simulink model "TorqueVect_HIL_CAN"  (R2022a)
settings: Solver=VariableStepAuto  StartTime=0.0  StopTime=300  RelTol=1e-3
PreLoadFcn:
  | run('Parameters\FSE_Parameters.m')
values from neighbouring files (symbols this model uses):
  Kd = 0;')    [open_carmaker_gui.m]
  Ki = 0    [open_carmaker_gui.m]
undefined symbols (not defined in the file or in its folder): BRegenEnabledButton, canChannel, CyalphaLookUp, efficiency, Fz_curve, Fz_scaling_long, gearR, izz, jw, kd, ki, Kp, kp, l_f, l_r, lambda, m, Mz_max, N, N_lat, N_long, P_max, pid_kd_lat, pid_kd_long, pid_ki_lat, pid_ki_long, pid_kp_lat, pid_kp_long, R_max, rw, steerR, T_i_max, TC_Decr_Gas, TC_Derivative, TC_Incr_Gas, TC_On, TC_Relay_Off, TC_Relay_On, tireCornerStiffness, Ts, TV_On, TV_Override, velocity_lookup, velocity_lookup_lat, y_ref, yrr_scaling
libraries: simulink x218, slpidlib x135, CarMaker4SL x73, TractionControlLibrary x13, canmsglib x11, canlib x10, TorqueVectoringLibrary x6, simulink_extras x4, PedalConversionLibrary x3, PowerControlLibrary x1
(part 17 of 26)

== system TorqueVect_HIL_CAN/CarMaker/IPG Vehicle/PowerTrain/PTControl Example/PTControl_ALL_CTRL_VC_REGEN/Subsystem/TC/TractionControlRL ==
  rSlipTarget : Inport
  rSlipMeasured : Inport  Port=2
  BEnableTC : Inport  Port=3
  P_TC : Inport  Port=4
  D_TC : Inport  Port=5
  I_TC : Inport  Port=6
  FF_TC : Inport  Port=7
  MMotorMax : Inport  Port=8
  MMotorRequest : Inport  Port=9
  If : If  NumInputs=2  IfExpression=u1 <= 0  ElseIfExpressions=u2 > u1
  If Action Subsystem : Subsystem  TreatAsAtomicUnit=on
  If Action Subsystem1 : Subsystem  TreatAsAtomicUnit=on
  If Action Subsystem2 : Subsystem  TreatAsAtomicUnit=on
  Merge : Merge  Inputs=3
  PID Controller : Subsystem  TreatAsAtomicUnit=on
  Product : Product
  Product1 : Product
  Saturation : Saturate  UpperLimit=1  LowerLimit=0
  Saturation1 : Saturate  UpperLimit=21  LowerLimit=0
  Saturation2 : Saturate  UpperLimit=0  LowerLimit=0
  Sum1 : Sum  Inputs=|-+
  Switch : Switch  Criteria=u2 > Threshold  SaturateOnIntegerOverflow=off  InputSameDT=off
  MMotorDemanded : Outport  VectorParamsAs1DForOutWhenUnconnected=off
  rSlipErrorRL : Outport  Port=2
  wires:
  rSlipTarget/1 -> Sum1/1
  MMotorRequest/1 -> Switch/2, If Action Subsystem/1(MMotorRequest), If/1, If Action Subsystem2/1(MMotorRequest)
  If/2 -> If Action Subsystem1/Action
  P_TC/1 -> PID Controller/3(Kp_TC)
  If Action Subsystem2/1(Out1) -> Merge/3
  FF_TC/1 -> Product/2
  Product/1 -> Sum1/2
  D_TC/1 -> PID Controller/4(Kd_TC)
  Saturation/1 -> rSlipErrorRL/1, PID Controller/1(rSlipError)
  If Action Subsystem/1(Out1) -> Merge/1
  Product1/1 -> Saturation/1
  If/3 -> If Action Subsystem2/Action
  BEnableTC/1 -> PID Controller/2(BEnable_TC), Product1/2
  If Action Subsystem1/1(Out1) -> Merge/2
  PID Controller/1(MMotorReduction) -> Saturation2/1, Saturation1/1
  I_TC/1 -> PID Controller/5(Ki_TC)
  Merge/1 -> MMotorDemanded/1
  Sum1/1 -> Product1/1
  If/1 -> If Action Subsystem/Action
  rSlipMeasured/1 -> Product/1
  MMotorMax/1 -> PID Controller/6(MMotorMax)
  Saturation2/1 -> Switch/3
  Saturation1/1 -> Switch/1
  Switch/1 -> If/2, If Action Subsystem2/2(In2)

== system TorqueVect_HIL_CAN/CarMaker/IPG Vehicle/PowerTrain/PTControl Example/PTControl_ALL_CTRL_VC_REGEN/Subsystem/TC/TractionControlRR ==
  rSlipTarget : Inport
  rSlipMeasured : Inport  Port=2
  BEnableTC : Inport  Port=3
  P_TC : Inport  Port=4
  D_TC : Inport  Port=5
  I_TC : Inport  Port=6
  FF_TC : Inport  Port=7
  MMotorMax : Inport  Port=8
  MMotorRequest : Inport  Port=9
  If : If  NumInputs=2  IfExpression=u1 <= 0  ElseIfExpressions=u2 > u1
  If Action Subsystem : Subsystem  TreatAsAtomicUnit=on
  If Action Subsystem1 : Subsystem  TreatAsAtomicUnit=on
  If Action Subsystem2 : Subsystem  TreatAsAtomicUnit=on
  Merge : Merge  Inputs=3
  PID Controller : Subsystem  TreatAsAtomicUnit=on
  Product : Product
  Product1 : Product
  Saturation : Saturate  UpperLimit=1  LowerLimit=0
  Saturation1 : Saturate  UpperLimit=21  LowerLimit=0
  Saturation2 : Saturate  UpperLimit=0  LowerLimit=0
  Sum1 : Sum  Inputs=|-+
  Switch : Switch  Criteria=u2 > Threshold  SaturateOnIntegerOverflow=off  InputSameDT=off
  MMotorDemanded : Outport  VectorParamsAs1DForOutWhenUnconnected=off
  rSlipErrorRR : Outport  Port=2
  wires:
  rSlipTarget/1 -> Sum1/1
  MMotorRequest/1 -> Switch/2, If Action Subsystem/1(MMotorRequest), If/1, If Action Subsystem2/1(MMotorRequest)
  If/2 -> If Action Subsystem1/Action
  P_TC/1 -> PID Controller/3(Kp_TC)
  If Action Subsystem2/1(Out1) -> Merge/3
  FF_TC/1 -> Product/2
  Product/1 -> Sum1/2
  D_TC/1 -> PID Controller/4(Kd_TC)
  Saturation/1 -> rSlipErrorRR/1, PID Controller/1(rSlipError)
  If Action Subsystem/1(Out1) -> Merge/1
  Product1/1 -> Saturation/1
  BEnableTC/1 -> PID Controller/2(BEnable_TC), Product1/2
  If Action Subsystem1/1(Out1) -> Merge/2
  PID Controller/1(MMotorReduction) -> Saturation2/1, Saturation1/1
  I_TC/1 -> PID Controller/5(Ki_TC)
  Merge/1 -> MMotorDemanded/1
  Sum1/1 -> Product1/1
  If/1 -> If Action Subsystem/Action
  rSlipMeasured/1 -> Product/1
  MMotorMax/1 -> PID Controller/6(MMotorMax)
  Saturation2/1 -> Switch/3
  Saturation1/1 -> Switch/1
  Switch/1 -> If/2, If Action Subsystem2/2(In2)
  If/3 -> If Action Subsystem2/Action

== system TorqueVect_HIL_CAN/CarMaker/IPG Vehicle/PowerTrain/PTControl Example/PTControl_ALL_CTRL_VC_REGEN/Subsystem/Torque Modification1/Torque Limit Check FL ==
  note: Checks for max value below 0 Nm when RC is acting
  note: Checks for min value when PC is acting
  MTorqueNewFL : Inport
  MDemandMotorFL : Inport  Port=2
  Max : MinMax  Function=max  Inputs=2
  Min : MinMax  Inputs=2
  Saturation : Saturate  UpperLimit=0  LowerLimit=-21
  Saturation1 : Saturate  UpperLimit=21  LowerLimit=0
  Switch : Switch  Criteria=u2 > Threshold  SaturateOnIntegerOverflow=off  InputSameDT=off
  MTorqueModFL : Outport
  wires:
  MDemandMotorFL/1 -> [MDemandMotorRL]
  [MDemandMotorRL] -> Min/1
  MTorqueNewFL/1 -> Saturation/1, Saturation1/1
  Switch/1 -> MTorqueModFL/1
  [MDemandMotorRL] -> Switch/2
  Min/1 -> Switch/1
  Max/1 -> Switch/3
  [MDemandMotorRL] -> ?
  Saturation/1 -> Max/1
  Saturation1/1 -> ?

== system TorqueVect_HIL_CAN/CarMaker/IPG Vehicle/PowerTrain/PTControl Example/PTControl_ALL_CTRL_VC_REGEN/Subsystem/Torque Modification1/Torque Limit Check FR ==
  note: Checks for max value below 0 Nm when RC is acting
  note: Checks for min value when PC is acting
  MTorqueNewFR : Inport
  MDemandMotorFR : Inport  Port=2
  Max : MinMax  Function=max  Inputs=2
  Min : MinMax  Inputs=2
  Saturation : Saturate  UpperLimit=0  LowerLimit=-21
  Saturation1 : Saturate  UpperLimit=21  LowerLimit=0
  Switch : Switch  Criteria=u2 > Threshold  SaturateOnIntegerOverflow=off  InputSameDT=off
  MTorqueModFR : Outport
  wires:
  MDemandMotorFR/1 -> [MDemandMotorRL]
  [MDemandMotorRL] -> Min/1
  MTorqueNewFR/1 -> Saturation/1, Saturation1/1
  Switch/1 -> MTorqueModFR/1
  [MDemandMotorRL] -> Switch/2
  Min/1 -> Switch/1
  Max/1 -> Switch/3
  [MDemandMotorRL] -> ?
  Saturation/1 -> Max/1
  Saturation1/1 -> ?

== system TorqueVect_HIL_CAN/CarMaker/IPG Vehicle/PowerTrain/PTControl Example/PTControl_ALL_CTRL_VC_REGEN/Subsystem/Torque Modification1/Torque Limit Check RL ==
  note: Checks for max value below 0 Nm when RC is acting
  note: Checks for min value when PC is acting
  MTorqueNewRL : Inport
  MDemandMotorRL : Inport  Port=2
  Max : MinMax  Function=max  Inputs=2
  Min : MinMax  Inputs=2
  Saturation : Saturate  UpperLimit=0  LowerLimit=-21
  Saturation1 : Saturate  UpperLimit=21  LowerLimit=0
  Switch : Switch  Criteria=u2 > Threshold  SaturateOnIntegerOverflow=off  InputSameDT=off
  MTorqueModRL : Outport
  wires:
  MDemandMotorRL/1 -> [MDemandMotorRL]
  [MDemandMotorRL] -> Min/1
  MTorqueNewRL/1 -> Saturation/1, Saturation1/1
  Switch/1 -> MTorqueModRL/1
  [MDemandMotorRL] -> Switch/2
  Min/1 -> Switch/1
  Max/1 -> Switch/3
  [MDemandMotorRL] -> ?
  Saturation/1 -> Max/1
  Saturation1/1 -> ?

== system TorqueVect_HIL_CAN/CarMaker/IPG Vehicle/PowerTrain/PTControl Example/PTControl_ALL_CTRL_VC_REGEN/Subsystem/Torque Modification1/Torque Limit Check RR ==
  note: Checks for max value below 0 Nm when RC is acting
  note: Checks for min value when PC is acting
  MTorqueNewRR : Inport
  MDemandMotorRR : Inport  Port=2
  Max : MinMax  Function=max  Inputs=2
  Min : MinMax  Inputs=2
  Saturation : Saturate  UpperLimit=0  LowerLimit=-21
  Saturation1 : Saturate  UpperLimit=21  LowerLimit=0
  Switch : Switch  Criteria=u2 > Threshold  SaturateOnIntegerOverflow=off  InputSameDT=off
  MTorqueModRR : Outport
  wires:
  MDemandMotorRR/1 -> [MDemandMotorRL]
  [MDemandMotorRL] -> Min/1
  MTorqueNewRR/1 -> Saturation/1, Saturation1/1
  Switch/1 -> MTorqueModRR/1
  [MDemandMotorRL] -> Switch/2
  Min/1 -> Switch/1
  Max/1 -> Switch/3
  [MDemandMotorRL] -> ?
  Saturation/1 -> Max/1
  Saturation1/1 -> ?

== system TorqueVect_HIL_CAN/CarMaker/IPG Vehicle/PowerTrain/PTControl Example/PTControl_ALL_CTRL_VC_REGEN/Subsystem/Torque Modification2/Torque Limit Check FL ==
  note: Checks for max value below 0 Nm when RC is acting
  note: Checks for min value when PC is acting
  MTorqueNewFL : Inport
  MDemandMotorFL : Inport  Port=2
  Max : MinMax  Function=max  Inputs=2
  Min : MinMax  Inputs=2
  Saturation : Saturate  UpperLimit=0  LowerLimit=-21
  Saturation1 : Saturate  UpperLimit=21  LowerLimit=0
  Switch : Switch  Criteria=u2 > Threshold  SaturateOnIntegerOverflow=off  InputSameDT=off
  MTorqueModFL : Outport
  wires:
  MDemandMotorFL/1 -> [MDemandMotorRL]
  [MDemandMotorRL] -> Min/1
  MTorqueNewFL/1 -> Saturation/1, Saturation1/1
  Switch/1 -> MTorqueModFL/1
  [MDemandMotorRL] -> Switch/2
  Min/1 -> Switch/1
  Max/1 -> Switch/3
  [MDemandMotorRL] -> Max/2
  Saturation/1 -> Max/1
  Saturation1/1 -> Min/2

== system TorqueVect_HIL_CAN/CarMaker/IPG Vehicle/PowerTrain/PTControl Example/PTControl_ALL_CTRL_VC_REGEN/Subsystem/Torque Modification2/Torque Limit Check FR ==
  note: Checks for max value below 0 Nm when RC is acting
  note: Checks for min value when PC is acting
  MTorqueNewFR : Inport
  MDemandMotorFR : Inport  Port=2
  Max : MinMax  Function=max  Inputs=2
  Min : MinMax  Inputs=2
  Saturation : Saturate  UpperLimit=0  LowerLimit=-21
  Saturation1 : Saturate  UpperLimit=21  LowerLimit=0
  Switch : Switch  Criteria=u2 > Threshold  SaturateOnIntegerOverflow=off  InputSameDT=off
  MTorqueModFR : Outport
  wires:
  MDemandMotorFR/1 -> [MDemandMotorRL]
  [MDemandMotorRL] -> Min/1
  MTorqueNewFR/1 -> Saturation/1, Saturation1/1
  Switch/1 -> MTorqueModFR/1
  [MDemandMotorRL] -> Switch/2
  Min/1 -> Switch/1
  Max/1 -> Switch/3
  [MDemandMotorRL] -> Max/2
  Saturation/1 -> Max/1
  Saturation1/1 -> Min/2

== system TorqueVect_HIL_CAN/CarMaker/IPG Vehicle/PowerTrain/PTControl Example/PTControl_ALL_CTRL_VC_REGEN/Subsystem/Torque Modification2/Torque Limit Check RL ==
  note: 6
  note: 6
  note: 18
  note: Checks for max value below 0 Nm when RC is acting
  note: Checks for min value when PC is acting
  MTorqueNewRL : Inport
  MDemandMotorRL : Inport  Port=2
  Max : MinMax  Function=max  Inputs=2
  Min : MinMax  Inputs=2
  Saturation : Saturate  UpperLimit=0  LowerLimit=-21
  Saturation1 : Saturate  UpperLimit=21  LowerLimit=0
  Switch : Switch  Criteria=u2 > Threshold  SaturateOnIntegerOverflow=off  InputSameDT=off
  MTorqueModRL : Outport
  wires:
  MDemandMotorRL/1 -> [MDemandMotorRL]
  [MDemandMotorRL] -> Min/1
  MTorqueNewRL/1 -> Saturation/1, Saturation1/1
  Switch/1 -> MTorqueModRL/1
  [MDemandMotorRL] -> Switch/2
  Min/1 -> Switch/1
  Max/1 -> Switch/3
  [MDemandMotorRL] -> Max/2
  Saturation/1 -> Max/1
  Saturation1/1 -> Min/2

== system TorqueVect_HIL_CAN/CarMaker/IPG Vehicle/PowerTrain/PTControl Example/PTControl_ALL_CTRL_VC_REGEN/Subsystem/Torque Modification2/Torque Limit Check RR ==
  note: Checks for max value below 0 Nm when RC is acting
  note: Checks for min value when PC is acting
  MTorqueNewRR : Inport
  MDemandMotorRR : Inport  Port=2
  Max : MinMax  Function=max  Inputs=2
  Min : MinMax  Inputs=2
  Saturation : Saturate  UpperLimit=0  LowerLimit=-21
  Saturation1 : Saturate  UpperLimit=21  LowerLimit=0
  Switch : Switch  Criteria=u2 > Threshold  SaturateOnIntegerOverflow=off  InputSameDT=off
  MTorqueModRR : Outport
  wires:
  MDemandMotorRR/1 -> [MDemandMotorRL]
  [MDemandMotorRL] -> Min/1
  MTorqueNewRR/1 -> Saturation/1, Saturation1/1
  Switch/1 -> MTorqueModRR/1
  [MDemandMotorRL] -> Switch/2
  Min/1 -> Switch/1
  Max/1 -> Switch/3
  [MDemandMotorRL] -> Max/2
  Saturation/1 -> Max/1
  Saturation1/1 -> Min/2

== system TorqueVect_HIL_CAN/CarMaker/IPG Vehicle/PowerTrain/PTControl Example/PTControl_ALL_CTRL_VC_REGEN/Subsystem/Torque Vectoring/FPID ==
  BEnable : Inport
  NTorqueMaxDelta : Inport  Port=2
  NTorqueMax : Inport  Port=3
  NTorqueAxle : Inport  Port=4
  aSlip : Inport  Port=5
  P_YR : Inport  Port=6
  D_YR : Inport  Port=7
  I_YR : Inport  Port=8
  Abs : Abs  SaturateOnIntegerOverflow=off
  Abs2 : Abs  SaturateOnIntegerOverflow=off
  Add : Sum  Inputs=+-
  Gain : Gain  Gain=0.5
  Gain1 : Gain  Gain=-1
  If Action Subsystem : Subsystem  TreatAsAtomicUnit=on
  Min : MinMax  Inputs=3
  PID Controller : slpidlib/PID Controller  Controller=PID  Form=Ideal  TimeDomain=Discrete-time  UseExternalTs=off  SampleTime=0.005  IntegratorMethod=Forward Euler  FilterMethod=Forward Euler  ControllerParametersSource=external  P=1  I=1  UseKiTs=on  D=0  N=100  UseFilter=off  TunerSelectOption=Transfer Function Based (PID Tuner App)  InitialConditionSource=internal  InitialConditionForIntegrator=0  InitialConditionForFilter=0  DifferentiatorICPrevScaledInput=0  ExternalReset=either  TrackingMode=off  Kt=1  LimitOutput=off  SatLimitsSource=external  UpperSaturationLimit=inf  LowerSaturationLimit=-inf  LinearizeAsGain=on  AntiWindupMode=clamping  Kb=1  POutMin=[]  POutMax=[]  IOutMin=[]  IOutMax=[]  DOutMin=[]  DOutMax=[]  NOutMin=[]  NOutMax=[]  SumOutMin=[]  SumOutMax=[]  SaturationOutMin=[]  SaturationOutMax=[]  PParamMin=[]  PParamMax=[]  IParamMin=[]  IParamMax=[]  DParamMin=[]  DParamMax=[]  NParamMin=[]  NParamMax=[]  KbParamMin=[]  KbParamMax=[]  KtParamMin=[]  KtParamMax=[]  KbOutMin=[]  KbOutMax=[]  KtOutMin=[]  KtOutMax=[]  IntegratorOutMin=[]  IntegratorOutMax=[]  FilterOutMin=[]  FilterOutMax=[]  SumI1OutMin=[]  SumI1OutMax=[]  SumI2OutMin=[]  SumI2OutMax=[]  SumI3OutMin=[]  SumI3OutMax=[]  SumI4OutMin=[]  SumI4OutMax=[]  SumDOutMin=[]  SumDOutMax=[]  DifferentiatorOutMin=[]  DifferentiatorOutMax=[]  FilterDiffOutCoefMin=[]  FilterDiffOutCoefMax=[]  ReciprocalOutMin=[]  ReciprocalOutMax=[]  SumDenOutMin=[]  SumDenOutMax=[]  SumNumOutMin=[]  SumNumOutMax=[]  DivideOutMin=[]  DivideOutMax=[]  UdiffTsProdOutMin=[]  UdiffTsProdOutMax=[]  NTsProdOutMin=[]  NTsProdOutMax=[]  UintegralTsProdOutMin=[]  UintegralTsProdOutMax=[]  UngainTsProdOutMin=[]  UngainTsProdOutMax=[]  ClampingZeroOutDataTypeStr=Inherit: Inherit via back propagation  ClampingZeroOutMin=[]  ClampingZeroOutMax=[]  FilterDenConstantOutDataTypeStr=Inherit: Inherit via back propagation  FilterDenConstantOutMin=[]  FilterDenConstantOutMax=[]  PCopyOutDataTypeStr=Inherit: Inherit via back propagation  PCopyOutMin=[]  PCopyOutMax=[]  NCopyOutDataTypeStr=Inherit: Inherit via back propagation  NCopyOutMin=[]  NCopyOutMax=[]  IntegratorContinuousStateAttributes=''  IntegratorStateMustResolveToSignalObject=off  IntegratorRTWStateStorageClass=Auto  FilterContinuousStateAttributes=''  FilterStateMustResolveToSignalObject=off  FilterRTWStateStorageClass=Auto  ParallelPVariant=Passthrough  IdealPVariant=ExternalParameters  IVariant=ExternalParameters  DVariant=ExternalParameters  IntegratorVariant=Discrete  SatVariant=Disabled  AWVariant=Passthrough  PCopyVariant=Disabled  TRVariant=Disabled  FdbkBlocksVariant=Forward  IdealPFdbkVariant=Disabled  SatFdbkVariant=Disabled  DerivativeFilterVariant=Differentiator  NVariant=Passthrough  NCopyVariant=Disabled_SignalSpec  FilterICVariant=InternalICsDifferentiator  IntegratorICVariant=InternalICs  ExternalResetVariant=ExternalReset  TRSumVariant=Passthrough  SumFdbkVariant=Disabled  SumVariant=Sum_PID  TsampFilterVariant=InternalTs  TsampNgainVariant=Passthrough  TsampIntegralVariant=Passthrough  ExternalSaturationOutDataTypeStr=Inherit: Same as second input  aMode=0
  Product : Product  Inputs=3
  Saturation Dynamic : simulink/Discontinuities/Saturation Dynamic  OutMin=[]  OutMax=[]  OutDataTypeStr=Inherit: Same as second input  OutDataType=fixdt(1, 16)  OutScaling=2^-10  DoSatur=off
  Saturation Dynamic1 : simulink/Discontinuities/Saturation Dynamic  OutMin=[]  OutMax=[]  OutDataTypeStr=Inherit: Same as second input  OutDataType=fixdt(1, 16)  OutScaling=2^-10  DoSatur=off
  Sign : Signum
  NTorqueLeftOut : Outport
  NTorqueRightOut : Outport  Port=2
  wires:
  I_YR/1 -> PID Controller/3
  [NTorqueWheel] -> If Action Subsystem/1(NTorqueWheel)
  aSlip/1 -> PID Controller/1
  NTorqueMax/1 -> [NTorqueMax]
  [NTorqueWheel] -> Abs/1
  NTorqueAxle/1 -> Gain/1
  [NTorqueMax] -> Add/1
  [BEnable] -> PID Controller/5
  Gain/1 -> [NTorqueWheel]
  P_YR/1 -> PID Controller/2
  [NTorqueMax] -> Saturation Dynamic1/1, Saturation Dynamic/1, Gain1/1
  [BEnable] -> Product/1
  Sign/1 -> Product/3
  [NTorqueDeltaTV] -> Abs2/1
  Abs/1 -> Add/2
  Product/1 -> If Action Subsystem/2(NTorqueDelta)
  Add/1 -> Min/2
  BEnable/1 -> [BEnable]
  Gain1/1 -> Saturation Dynamic1/3, Saturation Dynamic/3
  If Action Subsystem/2(NTorqueRightOut) -> Saturation Dynamic1/2  "NTorqueFROut"
  [NTorqueDeltaTV] -> Sign/1
  NTorqueMaxDelta/1 -> Min/1
  Min/1 -> Product/2
  If Action Subsystem/1(NTorqueLeftOut) -> Saturation Dynamic/2  "NTorqueFLOut"
  Abs2/1 -> Min/3
  D_YR/1 -> PID Controller/4
  PID Controller/1 -> [NTorqueDeltaTV]
  Saturation Dynamic1/1 -> NTorqueRightOut/1
  Saturation Dynamic/1 -> NTorqueLeftOut/1

== system TorqueVect_HIL_CAN/CarMaker/IPG Vehicle/PowerTrain/PTControl Example/PTControl_ALL_CTRL_VC_REGEN/Subsystem/Torque Vectoring/RPID ==
  BEnable : Inport
  NTorqueMaxDelta : Inport  Port=2
  NTorqueMax : Inport  Port=3
  NTorqueAxle : Inport  Port=4
  aSlip : Inport  Port=5
  P_YR : Inport  Port=6
  D_YR : Inport  Port=7
  I_YR : Inport  Port=8
  Abs : Abs  SaturateOnIntegerOverflow=off
  Abs2 : Abs  SaturateOnIntegerOverflow=off
  Add : Sum  Inputs=+-
  Gain : Gain  Gain=0.5
  Gain1 : Gain  Gain=-1
  If Action Subsystem : Subsystem  TreatAsAtomicUnit=on
  Min : MinMax  Inputs=3
  PID Controller : slpidlib/PID Controller  Controller=PID  Form=Ideal  TimeDomain=Discrete-time  UseExternalTs=off  SampleTime=0.005  IntegratorMethod=Forward Euler  FilterMethod=Forward Euler  ControllerParametersSource=external  P=1  I=1  UseKiTs=on  D=0  N=100  UseFilter=off  TunerSelectOption=Transfer Function Based (PID Tuner App)  InitialConditionSource=internal  InitialConditionForIntegrator=0  InitialConditionForFilter=0  DifferentiatorICPrevScaledInput=0  ExternalReset=either  TrackingMode=off  Kt=1  LimitOutput=off  SatLimitsSource=external  UpperSaturationLimit=inf  LowerSaturationLimit=-inf  LinearizeAsGain=on  AntiWindupMode=clamping  Kb=1  POutMin=[]  POutMax=[]  IOutMin=[]  IOutMax=[]  DOutMin=[]  DOutMax=[]  NOutMin=[]  NOutMax=[]  SumOutMin=[]  SumOutMax=[]  SaturationOutMin=[]  SaturationOutMax=[]  PParamMin=[]  PParamMax=[]  IParamMin=[]  IParamMax=[]  DParamMin=[]  DParamMax=[]  NParamMin=[]  NParamMax=[]  KbParamMin=[]  KbParamMax=[]  KtParamMin=[]  KtParamMax=[]  KbOutMin=[]  KbOutMax=[]  KtOutMin=[]  KtOutMax=[]  IntegratorOutMin=[]  IntegratorOutMax=[]  FilterOutMin=[]  FilterOutMax=[]  SumI1OutMin=[]  SumI1OutMax=[]  SumI2OutMin=[]  SumI2OutMax=[]  SumI3OutMin=[]  SumI3OutMax=[]  SumI4OutMin=[]  SumI4OutMax=[]  SumDOutMin=[]  SumDOutMax=[]  DifferentiatorOutMin=[]  DifferentiatorOutMax=[]  FilterDiffOutCoefMin=[]  FilterDiffOutCoefMax=[]  ReciprocalOutMin=[]  ReciprocalOutMax=[]  SumDenOutMin=[]  SumDenOutMax=[]  SumNumOutMin=[]  SumNumOutMax=[]  DivideOutMin=[]  DivideOutMax=[]  UdiffTsProdOutMin=[]  UdiffTsProdOutMax=[]  NTsProdOutMin=[]  NTsProdOutMax=[]  UintegralTsProdOutMin=[]  UintegralTsProdOutMax=[]  UngainTsProdOutMin=[]  UngainTsProdOutMax=[]  ClampingZeroOutDataTypeStr=Inherit: Inherit via back propagation  ClampingZeroOutMin=[]  ClampingZeroOutMax=[]  FilterDenConstantOutDataTypeStr=Inherit: Inherit via back propagation  FilterDenConstantOutMin=[]  FilterDenConstantOutMax=[]  PCopyOutDataTypeStr=Inherit: Inherit via back propagation  PCopyOutMin=[]  PCopyOutMax=[]  NCopyOutDataTypeStr=Inherit: Inherit via back propagation  NCopyOutMin=[]  NCopyOutMax=[]  IntegratorContinuousStateAttributes=''  IntegratorStateMustResolveToSignalObject=off  IntegratorRTWStateStorageClass=Auto  FilterContinuousStateAttributes=''  FilterStateMustResolveToSignalObject=off  FilterRTWStateStorageClass=Auto  ParallelPVariant=Passthrough  IdealPVariant=ExternalParameters  IVariant=ExternalParameters  DVariant=ExternalParameters  IntegratorVariant=Discrete  SatVariant=Disabled  AWVariant=Passthrough  PCopyVariant=Disabled  TRVariant=Disabled  FdbkBlocksVariant=Forward  IdealPFdbkVariant=Disabled  SatFdbkVariant=Disabled  DerivativeFilterVariant=Differentiator  NVariant=Passthrough  NCopyVariant=Disabled_SignalSpec  FilterICVariant=InternalICsDifferentiator  IntegratorICVariant=InternalICs  ExternalResetVariant=ExternalReset  TRSumVariant=Passthrough  SumFdbkVariant=Disabled  SumVariant=Sum_PID  TsampFilterVariant=InternalTs  TsampNgainVariant=Passthrough  TsampIntegralVariant=Passthrough  ExternalSaturationOutDataTypeStr=Inherit: Same as second input  aMode=0
  Product : Product  Inputs=3
  Saturation Dynamic : simulink/Discontinuities/Saturation Dynamic  OutMin=[]  OutMax=[]  OutDataTypeStr=Inherit: Same as second input  OutDataType=fixdt(1, 16)  OutScaling=2^-10  DoSatur=off
  Saturation Dynamic1 : simulink/Discontinuities/Saturation Dynamic  OutMin=[]  OutMax=[]  OutDataTypeStr=Inherit: Same as second input  OutDataType=fixdt(1, 16)  OutScaling=2^-10  DoSatur=off
  Sign : Signum
  NTorqueLeftOut : Outport
  NTorqueRightOut : Outport  Port=2
  wires:
  I_YR/1 -> PID Controller/3
  [NTorqueWheel] -> If Action Subsystem/1(NTorqueWheel)
  aSlip/1 -> PID Controller/1
  NTorqueMax/1 -> [NTorqueMax]
  [NTorqueWheel] -> Abs/1
  NTorqueAxle/1 -> Gain/1
  [NTorqueMax] -> Add/1
  [BEnable] -> PID Controller/5
  Gain/1 -> [NTorqueWheel]
  P_YR/1 -> PID Controller/2
  [NTorqueMax] -> Saturation Dynamic1/1, Saturation Dynamic/1, Gain1/1
  [BEnable] -> Product/1
  Sign/1 -> Product/3
  [NTorqueDeltaTV] -> Abs2/1
  Abs/1 -> Add/2
  Product/1 -> If Action Subsystem/2(NTorqueDelta)
  Add/1 -> Min/2
  BEnable/1 -> [BEnable]
  Gain1/1 -> Saturation Dynamic1/3, Saturation Dynamic/3
  If Action Subsystem/2(NTorqueRightOut) -> Saturation Dynamic1/2  "NTorqueRROut"
  [NTorqueDeltaTV] -> Sign/1
  NTorqueMaxDelta/1 -> Min/1
  Min/1 -> Product/2
  If Action Subsystem/1(NTorqueLeftOut) -> Saturation Dynamic/2  "NTorqueRLOut"
  Abs2/1 -> Min/3
  D_YR/1 -> PID Controller/4
  PID Controller/1 -> [NTorqueDeltaTV]
  Saturation Dynamic1/1 -> NTorqueRightOut/1
  Saturation Dynamic/1 -> NTorqueLeftOut/1

== system TorqueVect_HIL_CAN/CarMaker/IPG Vehicle/PowerTrain/PTControl Example/PTControl_ALL_CTRL_VC_REGEN/Subsystem1/PowerControl/PC PID ==
  PError : Inport
  P_PC : Inport  Port=2
  D_PC : Inport  Port=3
  I_PC : Inport  Port=4
  ResetPID_PC : Inport  Port=5
  MMotorMax : Inport  Port=6
  Constant : Constant  Value=0
  Gain : Gain  Gain=4
  Gain1 : Gain  Gain=0.01
  PID Controller : slpidlib/PID Controller  Controller=PID  Form=Ideal  TimeDomain=Discrete-time  UseExternalTs=off  SampleTime=0.005  IntegratorMethod=Backward Euler  FilterMethod=Forward Euler  ControllerParametersSource=external  P=1  I=1  UseKiTs=on  D=0  N=100  UseFilter=off  TunerSelectOption=Transfer Function Based (PID Tuner App)  InitialConditionSource=internal  InitialConditionForIntegrator=0  InitialConditionForFilter=0  DifferentiatorICPrevScaledInput=0  ExternalReset=rising  TrackingMode=off  Kt=1  LimitOutput=on  SatLimitsSource=external  UpperSaturationLimit=84  LowerSaturationLimit=0  LinearizeAsGain=on  AntiWindupMode=clamping  Kb=2  SaturateOnIntegerOverflow=on  POutMin=[]  POutMax=[]  IOutMin=[]  IOutMax=[]  DOutMin=[]  DOutMax=[]  NOutMin=[]  NOutMax=[]  SumOutMin=[]  SumOutMax=[]  SaturationOutMin=[]  SaturationOutMax=[]  PParamMin=[]  PParamMax=[]  IParamMin=[]  IParamMax=[]  DParamMin=[]  DParamMax=[]  NParamMin=[]  NParamMax=[]  KbParamMin=[]  KbParamMax=[]  KtParamMin=[]  KtParamMax=[]  KbOutMin=[]  KbOutMax=[]  KtOutMin=[]  KtOutMax=[]  IntegratorOutMin=[]  IntegratorOutMax=[]  FilterOutMin=[]  FilterOutMax=[]  SumI1OutMin=[]  SumI1OutMax=[]  SumI2OutMin=[]  SumI2OutMax=[]  SumI3OutMin=[]  SumI3OutMax=[]  SumI4OutMin=[]  SumI4OutMax=[]  SumDOutMin=[]  SumDOutMax=[]  DifferentiatorOutMin=[]  DifferentiatorOutMax=[]  FilterDiffOutCoefMin=[]  FilterDiffOutCoefMax=[]  ReciprocalOutMin=[]  ReciprocalOutMax=[]  SumDenOutMin=[]  SumDenOutMax=[]  SumNumOutMin=[]  SumNumOutMax=[]  DivideOutMin=[]  DivideOutMax=[]  UdiffTsProdOutMin=[]  UdiffTsProdOutMax=[]  NTsProdOutMin=[]  NTsProdOutMax=[]  UintegralTsProdOutMin=[]  UintegralTsProdOutMax=[]  UngainTsProdOutMin=[]  UngainTsProdOutMax=[]  ClampingZeroOutDataTypeStr=Inherit: Inherit via back propagation  ClampingZeroOutMin=[]  ClampingZeroOutMax=[]  FilterDenConstantOutDataTypeStr=Inherit: Inherit via back propagation  FilterDenConstantOutMin=[]  FilterDenConstantOutMax=[]  PCopyOutDataTypeStr=Inherit: Inherit via back propagation  PCopyOutMin=[]  PCopyOutMax=[]  NCopyOutDataTypeStr=Inherit: Inherit via back propagation  NCopyOutMin=[]  NCopyOutMax=[]  IntegratorContinuousStateAttributes=''  IntegratorStateMustResolveToSignalObject=off  IntegratorRTWStateStorageClass=Auto  FilterContinuousStateAttributes=''  FilterStateMustResolveToSignalObject=off  FilterRTWStateStorageClass=Auto  ParallelPVariant=Passthrough  IdealPVariant=ExternalParameters  IVariant=ExternalParameters  DVariant=ExternalParameters  IntegratorVariant=Discrete  SatVariant=External  AWVariant=DiscClampingIdeal  PCopyVariant=ExternalParamsIdeal  TRVariant=Disabled  FdbkBlocksVariant=Feedback  IdealPFdbkVariant=ExternalParameters  SatFdbkVariant=Passthrough  DerivativeFilterVariant=Differentiator  NVariant=Passthrough  NCopyVariant=Disabled_SignalSpec  FilterICVariant=InternalICsDifferentiator  IntegratorICVariant=InternalICs  ExternalResetVariant=ExternalReset  TRSumVariant=Passthrough  SumFdbkVariant=Enabled  SumVariant=Sum_PID  TsampFilterVariant=InternalTs  TsampNgainVariant=Passthrough  TsampIntegralVariant=Passthrough  ExternalSaturationOutDataTypeStr=Inherit: Same as second input  aMode=0
  TrqReductionTotal : Outport
  wires:
  PID Controller/1 -> TrqReductionTotal/1  "control input delta_P"
  D_PC/1 -> PID Controller/4
  P_PC/1 -> PID Controller/2
  I_PC/1 -> PID Controller/3
  ResetPID_PC/1 -> PID Controller/5
  MMotorMax/1 -> Gain/1
  Gain/1 -> PID Controller/6
  Gain1/1 -> PID Controller/1
  PError/1 -> Gain1/1
  Constant/1 -> PID Controller/7

== system TorqueVect_HIL_CAN/CarMaker/IPG Vehicle/PowerTrain/PTControl Example/PTControl_ALL_CTRL_VC_REGEN/Subsystem1/PowerControl/PID1 ==
  PError : Inport
  PRegenError : Inport  Port=2
  P_PC : Inport  Port=3
  D_PC : Inport  Port=4
  I_PC : Inport  Port=5
  ResetPID_PC : Inport  Port=6
  MMotorMax : Inport  Port=7
  BRegenEnabled : Inport  Port=8
  rThrottlePedal : Inport  Port=9
  AND : Logic  IconShape=distinctive  AllPortsSameDT=off  OutDataTypeStr=boolean
  Add : Sum
  Compare To Constant : simulink/Logic and Bit Operations/Compare To Constant  relop=<=  const=0.1  OutDataTypeStr=boolean
  Constant : Constant  Value=0
  Gain : Gain  Gain=4
  Gain1 : Gain  Gain=0.01
  Gain2 : Gain  Gain=-1
  PID Controller : slpidlib/PID Controller  Controller=PID  Form=Ideal  TimeDomain=Discrete-time  UseExternalTs=off  SampleTime=0.005  IntegratorMethod=Backward Euler  FilterMethod=Forward Euler  ControllerParametersSource=external  P=1  I=1  UseKiTs=on  D=0  N=100  UseFilter=off  TunerSelectOption=Transfer Function Based (PID Tuner App)  InitialConditionSource=internal  InitialConditionForIntegrator=0  InitialConditionForFilter=0  DifferentiatorICPrevScaledInput=0  ExternalReset=rising  TrackingMode=off  Kt=1  LimitOutput=on  SatLimitsSource=external  UpperSaturationLimit=84  LowerSaturationLimit=0  LinearizeAsGain=on  AntiWindupMode=clamping  Kb=2  SaturateOnIntegerOverflow=on  POutMin=[]  POutMax=[]  IOutMin=[]  IOutMax=[]  DOutMin=[]  DOutMax=[]  NOutMin=[]  NOutMax=[]  SumOutMin=[]  SumOutMax=[]  SaturationOutMin=[]  SaturationOutMax=[]  PParamMin=[]  PParamMax=[]  IParamMin=[]  IParamMax=[]  DParamMin=[]  DParamMax=[]  NParamMin=[]  NParamMax=[]  KbParamMin=[]  KbParamMax=[]  KtParamMin=[]  KtParamMax=[]  KbOutMin=[]  KbOutMax=[]  KtOutMin=[]  KtOutMax=[]  IntegratorOutMin=[]  IntegratorOutMax=[]  FilterOutMin=[]  FilterOutMax=[]  SumI1OutMin=[]  SumI1OutMax=[]  SumI2OutMin=[]  SumI2OutMax=[]  SumI3OutMin=[]  SumI3OutMax=[]  SumI4OutMin=[]  SumI4OutMax=[]  SumDOutMin=[]  SumDOutMax=[]  DifferentiatorOutMin=[]  DifferentiatorOutMax=[]  FilterDiffOutCoefMin=[]  FilterDiffOutCoefMax=[]  ReciprocalOutMin=[]  ReciprocalOutMax=[]  SumDenOutMin=[]  SumDenOutMax=[]  SumNumOutMin=[]  SumNumOutMax=[]  DivideOutMin=[]  DivideOutMax=[]  UdiffTsProdOutMin=[]  UdiffTsProdOutMax=[]  NTsProdOutMin=[]  NTsProdOutMax=[]  UintegralTsProdOutMin=[]  UintegralTsProdOutMax=[]  UngainTsProdOutMin=[]  UngainTsProdOutMax=[]  ClampingZeroOutDataTypeStr=Inherit: Inherit via back propagation  ClampingZeroOutMin=[]  ClampingZeroOutMax=[]  FilterDenConstantOutDataTypeStr=Inherit: Inherit via back propagation  FilterDenConstantOutMin=[]  FilterDenConstantOutMax=[]  PCopyOutDataTypeStr=Inherit: Inherit via back propagation  PCopyOutMin=[]  PCopyOutMax=[]  NCopyOutDataTypeStr=Inherit: Inherit via back propagation  NCopyOutMin=[]  NCopyOutMax=[]  IntegratorContinuousStateAttributes=''  IntegratorStateMustResolveToSignalObject=off  IntegratorRTWStateStorageClass=Auto  FilterContinuousStateAttributes=''  FilterStateMustResolveToSignalObject=off  FilterRTWStateStorageClass=Auto  ParallelPVariant=Passthrough  IdealPVariant=ExternalParameters  IVariant=ExternalParameters  DVariant=ExternalParameters  IntegratorVariant=Discrete  SatVariant=External  AWVariant=DiscClampingIdeal  PCopyVariant=ExternalParamsIdeal  TRVariant=Disabled  FdbkBlocksVariant=Feedback  IdealPFdbkVariant=ExternalParameters  SatFdbkVariant=Passthrough  DerivativeFilterVariant=Differentiator  NVariant=Passthrough  NCopyVariant=Disabled_SignalSpec  FilterICVariant=InternalICsDifferentiator  IntegratorICVariant=InternalICs  ExternalResetVariant=ExternalReset  TRSumVariant=Passthrough  SumFdbkVariant=Enabled  SumVariant=Sum_PID  TsampFilterVariant=InternalTs  TsampNgainVariant=Passthrough  TsampIntegralVariant=Passthrough  ExternalSaturationOutDataTypeStr=Inherit: Same as second input  aMode=0
  Switch : Switch  Criteria=u2 > Threshold  SaturateOnIntegerOverflow=off  InputSameDT=off
  TrqReductionTotal : Outport
  wires:
  PID Controller/1 -> TrqReductionTotal/1  "control input delta_P"
  D_PC/1 -> PID Controller/4
  P_PC/1 -> PID Controller/2
  I_PC/1 -> PID Controller/3
  ResetPID_PC/1 -> PID Controller/5
  MMotorMax/1 -> Gain/1
  Gain/1 -> Gain2/1, PID Controller/6
  Gain1/1 -> PID Controller/1
  Add/1 -> Gain1/1
  PError/1 -> Add/1
  PRegenError/1 -> Add/2
  rThrottlePedal/1 -> Compare To Constant/1
  BRegenEnabled/1 -> AND/1
  Compare To Constant/1 -> AND/2
  AND/1 -> Switch/2
  Switch/1 -> PID Controller/7
  Constant/1 -> Switch/3
  Gain2/1 -> Switch/1

== system TorqueVect_HIL_CAN/CarMaker/IPG Vehicle/PowerTrain/PTControl Example/PTControl_ALL_CTRL_VC_REGEN/Subsystem1/PowerControl/PowerError ==
  PPositiveTotal : Inport  Unit=W  PortDimensions=1
      settings: AttributesFormatString=%<Unit>
  FF_PC : Inport  Port=2
  PLimit : Inport  Port=3  OutMin=0  OutMax=80000  Unit=W  PortDimensions=1
      settings: AttributesFormatString=[%<OutMin>, %<OutMax>] %<Unit>
  Product5 : Product
  Saturation2 : Saturate  UpperLimit=250000  LowerLimit=0
      settings: AttributesFormatString=[%<LowerLimit>, %<UpperLimit>] W
  Subtract2 : Sum  Inputs=+-
  PError : Outport  Unit=W  PortDimensions=1
      settings: AttributesFormatString=%<Unit>
  wires:
  FF_PC/1 -> Product5/2
  Subtract2/1 -> Saturation2/1
  PLimit/1 -> Subtract2/2
  PPositiveTotal/1 -> Product5/1
  Saturation2/1 -> PError/1  "power error"
  Product5/1 -> Subtract2/1

== system TorqueVect_HIL_CAN/CarMaker/IPG Vehicle/PowerTrain/PTControl Example/PTControl_ALL_CTRL_VC_REGEN/Subsystem1/PowerControl/RC PID ==
  PRegenError : Inport
  P_RC : Inport  Port=2
  D_RC : Inport  Port=3
  I_RC : Inport  Port=4
  ResetPID_RC : Inport  Port=5
  MRegenMotorMax : Inport  Port=6
  Constant : Constant  Value=0
  Gain : Gain  Gain=-4
  Gain1 : Gain  Gain=0.01
  PID Controller : slpidlib/PID Controller  Controller=PID  Form=Ideal  TimeDomain=Discrete-time  UseExternalTs=off  SampleTime=0.005  IntegratorMethod=Backward Euler  FilterMethod=Forward Euler  ControllerParametersSource=external  P=1  I=1  UseKiTs=on  D=0  N=100  UseFilter=off  TunerSelectOption=Transfer Function Based (PID Tuner App)  InitialConditionSource=internal  InitialConditionForIntegrator=0  InitialConditionForFilter=0  DifferentiatorICPrevScaledInput=0  ExternalReset=level  TrackingMode=off  Kt=1  LimitOutput=on  SatLimitsSource=external  UpperSaturationLimit=84  LowerSaturationLimit=0  LinearizeAsGain=on  AntiWindupMode=clamping  Kb=2  SaturateOnIntegerOverflow=on  POutMin=[]  POutMax=[]  IOutMin=[]  IOutMax=[]  DOutMin=[]  DOutMax=[]  NOutMin=[]  NOutMax=[]  SumOutMin=[]  SumOutMax=[]  SaturationOutMin=[]  SaturationOutMax=[]  PParamMin=[]  PParamMax=[]  IParamMin=[]  IParamMax=[]  DParamMin=[]  DParamMax=[]  NParamMin=[]  NParamMax=[]  KbParamMin=[]  KbParamMax=[]  KtParamMin=[]  KtParamMax=[]  KbOutMin=[]  KbOutMax=[]  KtOutMin=[]  KtOutMax=[]  IntegratorOutMin=[]  IntegratorOutMax=[]  FilterOutMin=[]  FilterOutMax=[]  SumI1OutMin=[]  SumI1OutMax=[]  SumI2OutMin=[]  SumI2OutMax=[]  SumI3OutMin=[]  SumI3OutMax=[]  SumI4OutMin=[]  SumI4OutMax=[]  SumDOutMin=[]  SumDOutMax=[]  DifferentiatorOutMin=[]  DifferentiatorOutMax=[]  FilterDiffOutCoefMin=[]  FilterDiffOutCoefMax=[]  ReciprocalOutMin=[]  ReciprocalOutMax=[]  SumDenOutMin=[]  SumDenOutMax=[]  SumNumOutMin=[]  SumNumOutMax=[]  DivideOutMin=[]  DivideOutMax=[]  UdiffTsProdOutMin=[]  UdiffTsProdOutMax=[]  NTsProdOutMin=[]  NTsProdOutMax=[]  UintegralTsProdOutMin=[]  UintegralTsProdOutMax=[]  UngainTsProdOutMin=[]  UngainTsProdOutMax=[]  ClampingZeroOutDataTypeStr=Inherit: Inherit via back propagation  ClampingZeroOutMin=[]  ClampingZeroOutMax=[]  FilterDenConstantOutDataTypeStr=Inherit: Inherit via back propagation  FilterDenConstantOutMin=[]  FilterDenConstantOutMax=[]  PCopyOutDataTypeStr=Inherit: Inherit via back propagation  PCopyOutMin=[]  PCopyOutMax=[]  NCopyOutDataTypeStr=Inherit: Inherit via back propagation  NCopyOutMin=[]  NCopyOutMax=[]  IntegratorContinuousStateAttributes=''  IntegratorStateMustResolveToSignalObject=off  IntegratorRTWStateStorageClass=Auto  FilterContinuousStateAttributes=''  FilterStateMustResolveToSignalObject=off  FilterRTWStateStorageClass=Auto  ParallelPVariant=Passthrough  IdealPVariant=ExternalParameters  IVariant=ExternalParameters  DVariant=ExternalParameters  IntegratorVariant=Discrete  SatVariant=External  AWVariant=DiscClampingIdeal  PCopyVariant=ExternalParamsIdeal  TRVariant=Disabled  FdbkBlocksVariant=Feedback  IdealPFdbkVariant=ExternalParameters  SatFdbkVariant=Passthrough  DerivativeFilterVariant=Differentiator  NVariant=Passthrough  NCopyVariant=Disabled_SignalSpec  FilterICVariant=InternalICsDifferentiator  IntegratorICVariant=InternalICs  ExternalResetVariant=ExternalReset  TRSumVariant=Passthrough  SumFdbkVariant=Enabled  SumVariant=Sum_PID  TsampFilterVariant=InternalTs  TsampNgainVariant=Passthrough  TsampIntegralVariant=Passthrough  ExternalSaturationOutDataTypeStr=Inherit: Same as second input  aMode=0
  RegenTrqReductionTotal : Outport
  wires:
  PID Controller/1 -> RegenTrqReductionTotal/1  "control input delta_P"
  D_RC/1 -> PID Controller/4
  P_RC/1 -> PID Controller/2
  I_RC/1 -> PID Controller/3
  ResetPID_RC/1 -> PID Controller/5
  MRegenMotorMax/1 -> Gain/1
  Gain1/1 -> PID Controller/1
  PRegenError/1 -> Gain1/1
  Gain/1 -> PID Controller/7
  Constant/1 -> PID Controller/6

== system TorqueVect_HIL_CAN/CarMaker/IPG Vehicle/PowerTrain/PTControl Example/PTControl_ALL_CTRL_VC_REGEN/Subsystem1/PowerControl/RegenError ==
  PackVoltage : Inport
  Current : Inport  Port=2
  CurrentLimit : Inport  Port=3
  FF_RC : Inport  Port=4
  rThrottle : Inport  Port=5
  BRegenEnabled : Inport  Port=6
  Product : Product
  Product1 : Product  Inputs=3
  Product6 : Product
  Saturation : Saturate  UpperLimit=0  LowerLimit=-250000
  Saturation7 : Saturate  UpperLimit=0  LowerLimit=-250000
      settings: AttributesFormatString=[%<LowerLimit>, %<UpperLimit>] W
  Subtract1 : Sum  Inputs=+-
  PRegenError : Outport  Unit=W  PortDimensions=1
      settings: AttributesFormatString=%<Unit>
  wires:
  Saturation/1 -> Subtract1/2
  CurrentLimit/1 -> Product/2
  rThrottle/1 -> Product/1
  Product/1 -> Saturation/1
  Subtract1/1 -> Saturation7/1
  Current/1 -> Product6/1
  Product6/1 -> Subtract1/1
  FF_RC/1 -> Product6/2
  Product1/1 -> PRegenError/1
  Saturation7/1 -> Product1/1  "regen error"
  BRegenEnabled/1 -> Product1/3
  PackVoltage/1 -> Product1/2

== system TorqueVect_HIL_CAN/CarMaker/IPG Vehicle/PowerTrain/PTControl Example/PTControl_ALL_CTRL_VC_REGEN/Subsystem1/PowerControl/ResetPID_PC ==
  note: Resets when the pedal is below pos torque demand and there is still a reduction by the PID
  note: Resets when the pedal is in the idle zone [8-11%]
  rThrottlePedal : Inport
  PReductionTotal : Inport  Port=2
  AND : Logic  IconShape=distinctive  AllPortsSameDT=off  OutDataTypeStr=boolean
  AND1 : Logic  Inputs=3  IconShape=distinctive  AllPortsSameDT=off  OutDataTypeStr=boolean
  Compare To Constant1 : simulink/Logic and Bit Operations/Compare To Constant  relop=<=  const=0.1  OutDataTypeStr=boolean
  Compare To Constant2 : simulink/Logic and Bit Operations/Compare To Constant  relop=<=  const=0.11  OutDataTypeStr=boolean
  Compare To Constant3 : simulink/Logic and Bit Operations/Compare To Constant  relop=>=  const=0.08  OutDataTypeStr=boolean
  Compare To Constant4 : simulink/Logic and Bit Operations/Compare To Constant  relop=>  const=0  OutDataTypeStr=boolean
  Detect Fall Negative1 : simulink/Logic and Bit Operations/Detect Fall Negative  vinit=0  OutDataTypeStr=boolean
      settings: SourceProductBaseCode=SL
  Discrete Derivative1 : simulink/Discrete/Discrete Derivative  gainval=1.0  ICPrevScaledInput=0.0  OutMin=[]  OutMax=[]  OutDataType=fixdt(1, 16)  OutScaling=2^-10  DoSatur=off
  OR : Logic  Operator=OR  IconShape=distinctive  AllPortsSameDT=off  OutDataTypeStr=boolean
  ResetPID_PC : Outport
  wires:
  rThrottlePedal/1 -> Compare To Constant1/1, Compare To Constant3/1, Compare To Constant2/1, Discrete Derivative1/1
  Discrete Derivative1/1 -> Detect Fall Negative1/1
  Detect Fall Negative1/1 -> AND1/2  "accel_pedal_falling_or"
  Compare To Constant2/1 -> AND1/1
  Compare To Constant3/1 -> AND1/3
  OR/1 -> ResetPID_PC/1
  Compare To Constant1/1 -> AND/1
  Compare To Constant4/1 -> AND/2
  PReductionTotal/1 -> Compare To Constant4/1
  AND1/1 -> OR/1
  AND/1 -> OR/2

== system TorqueVect_HIL_CAN/CarMaker/IPG Vehicle/PowerTrain/PTControl Example/PTControl_ALL_CTRL_VC_REGEN/Subsystem1/PowerControl/ResetPID_RC ==
  note: Resets when the pedal is above regen torque demand and there is still a reaction by the PID
  note: Resets when the pedal is in the idle zone [8-11%]
  note: Resets when regen becomes disabled
  rThrottlePedal : Inport
  RegenTrqReductionTotal : Inport  Port=2
  BRegenEnabled : Inport  Port=3
  Current : Inport  Port=4
  AND : Logic  IconShape=distinctive  AllPortsSameDT=off  OutDataTypeStr=boolean
  AND1 : Logic  Inputs=3  IconShape=distinctive  AllPortsSameDT=off  OutDataTypeStr=boolean
  Compare To Constant : simulink/Logic and Bit Operations/Compare To Constant  relop===  const=0  OutDataTypeStr=boolean
  Compare To Constant1 : simulink/Logic and Bit Operations/Compare To Constant  relop=>=  const=0.07  OutDataTypeStr=boolean
  Compare To Constant2 : simulink/Logic and Bit Operations/Compare To Constant  relop=<=  const=0.1  OutDataTypeStr=boolean
  Compare To Constant3 : simulink/Logic and Bit Operations/Compare To Constant  relop=>=  const=0.07  OutDataTypeStr=boolean
  Compare To Constant4 : simulink/Logic and Bit Operations/Compare To Constant  relop=<  const=0  OutDataTypeStr=boolean
  Compare To Constant5 : simulink/Logic and Bit Operations/Compare To Constant  relop=>=  const=0  OutDataTypeStr=boolean
  Detect Fall Negative : simulink/Logic and Bit Operations/Detect Fall Negative  vinit=0  OutDataTypeStr=boolean
      settings: SourceProductBaseCode=SL
  Detect Rise Positive : simulink/Logic and Bit Operations/Detect Rise Positive  vinit=0  OutDataTypeStr=boolean
  Discrete Derivative1 : simulink/Discrete/Discrete Derivative  gainval=1.0  ICPrevScaledInput=0.0  OutMin=[]  OutMax=[]  OutDataType=fixdt(1, 16)  OutScaling=2^-10  DoSatur=off
  OR : Logic  Operator=OR  Inputs=4  IconShape=distinctive  AllPortsSameDT=off  OutDataTypeStr=boolean
  OR1 : Logic  Operator=OR  IconShape=distinctive  AllPortsSameDT=off  OutDataTypeStr=boolean
  ResetPID_RC : Outport
  wires:
  rThrottlePedal/1 -> Compare To Constant1/1, Compare To Constant3/1, Compare To Constant2/1, Discrete Derivative1/1
  Discrete Derivative1/1 -> Detect Rise Positive/1
  Detect Rise Positive/1 -> AND1/2  "accel_pedal_rising_or"
  Compare To Constant2/1 -> AND1/1
  Compare To Constant3/1 -> AND1/3
  OR/1 -> ResetPID_RC/1
  Compare To Constant1/1 -> AND/1
  Compare To Constant4/1 -> AND/2
  RegenTrqReductionTotal/1 -> Compare To Constant4/1
  AND/1 -> OR/3
  AND1/1 -> OR/2
  BRegenEnabled/1 -> Compare To Constant/1, Detect Fall Negative/1
  Detect Fall Negative/1 -> OR1/2
  Compare To Constant/1 -> OR1/1
  OR1/1 -> OR/1
  Current/1 -> Compare To Constant5/1
  Compare To Constant5/1 -> OR/4

== system TorqueVect_HIL_CAN/CarMaker/IPG Vehicle/PowerTrain/PTControl Example/PTControl_ALL_CTRL_VC_REGEN/Subsystem1/PowerControl/Subsystem ==
  TrqReductionTotal : Inport
  rSplitF : Inport  Port=2
  Constant : Constant
  Product : Product
  Sum : Sum  Inputs=|+-
  Sum1 : Sum  Inputs=|-+
  TrqReductionR : Outport
  TrqReductionF : Outport  Port=2
  wires:
  TrqReductionTotal/1 -> Product/1, Sum/1
  Product/1 -> TrqReductionF/1, Sum/2
  Sum/1 -> TrqReductionR/1
  rSplitF/1 -> Sum1/1
  Constant/1 -> Sum1/2
  Sum1/1 -> Product/2

== system TorqueVect_HIL_CAN/CarMaker/IPG Vehicle/PowerTrain/PTControl Example/PTControl_ALL_CTRL_VC_REGEN/Subsystem1/PowerControl/TotalPower ==
  MMotorFL : Inport  OutMin=-42  OutMax=42  Unit=N*m  PortDimensions=1
      settings: AttributesFormatString=[%<OutMin>, %<OutMax>] %<Unit>
  nMotorFL : Inport  Port=2  OutMin=-3000  OutMax=3000  Unit=rad/s  PortDimensions=1
      settings: AttributesFormatString=[%<OutMin>, %<OutMax>] %<Unit>
  MMotorFR : Inport  Port=3  OutMin=-42  OutMax=42  Unit=N*m  PortDimensions=1
      settings: AttributesFormatString=[%<OutMin>, %<OutMax>] %<Unit>
  nMotorFR : Inport  Port=4  OutMin=-3000  OutMax=3000  Unit=rad/s  PortDimensions=1
      settings: AttributesFormatString=[%<OutMin>, %<OutMax>] %<Unit>
  MMotorRL : Inport  Port=5  OutMin=-42  OutMax=42  Unit=N*m  PortDimensions=1
      settings: AttributesFormatString=[%<OutMin>, %<OutMax>] %<Unit>
  nMotorRL : Inport  Port=6  OutMin=-3000  OutMax=3000  Unit=rad/s  PortDimensions=1
      settings: AttributesFormatString=[%<OutMin>, %<OutMax>] %<Unit>
  MMotorRR : Inport  Port=7  OutMin=-42  OutMax=42  Unit=N*m  PortDimensions=1
      settings: AttributesFormatString=[%<OutMin>, %<OutMax>] %<Unit>
  nMotorRR : Inport  Port=8  OutMin=-3000  OutMax=3000  Unit=rad/s  PortDimensions=1
      settings: AttributesFormatString=[%<OutMin>, %<OutMax>] %<Unit>
  PMeasured : Inport  Port=9  OutMin=-250000  OutMax=250000  Unit=W  PortDimensions=1
      settings: AttributesFormatString=[%<OutMin>, %<OutMax>] %<Unit>
  BMeasuredEnable : Inport  Port=10  OutMin=0  OutMax=1  PortDimensions=1
      settings: AttributesFormatString=[%<OutMin> / %<OutMax>]
  Product{2,7..9} (4 alike) : Product
  Saturation{1,3..5} (4 alike) : Saturate  UpperLimit=250000  LowerLimit=0
  Sum3 : Sum  Inputs=++++
  Switch : Switch  Threshold=1  SaturateOnIntegerOverflow=off  InputSameDT=off
  PPositiveTotal : Outport  OutMin=0  OutMax=250000  Unit=W  PortDimensions=1
      settings: AttributesFormatString=[%<OutMin>, %<OutMax>] %<Unit>
  wires:
  MMotorRR/1 -> Product9/2
  nMotorRR/1 -> Product9/1
  nMotorRL/1 -> Product8/2
  MMotorRL/1 -> Product8/1
  nMotorFR/1 -> Product7/2
  MMotorFR/1 -> Product7/1
  nMotorFL/1 -> Product2/2
  MMotorFL/1 -> Product2/1
  Product9/1 -> Saturation5/1
  Product8/1 -> Saturation4/1
  Product7/1 -> Saturation3/1
  BMeasuredEnable/1 -> Switch/2
  PMeasured/1 -> Switch/1
  Switch/1 -> PPositiveTotal/1
  Saturation1/1 -> Sum3/1
  Saturation4/1 -> Sum3/3
  Product2/1 -> Saturation1/1
  Saturation5/1 -> Sum3/4
  Sum3/1 -> Switch/3  "tot_powerrrr_PC"
  Saturation3/1 -> Sum3/2

== system TorqueVect_HIL_CAN/CarMaker/IPG Vehicle/PowerTrain/PTControl Example/PTControl_ALL_CTRL_VC_REGEN/Subsystem1/PowerControl1/PID ==
  PError : Inport
  P_PC : Inport  Port=2
  D_PC : Inport  Port=3
  I_PC : Inport  Port=4
  ResetPID_PC : Inport  Port=5
  PID Controller : slpidlib/PID Controller  Controller=PID  Form=Parallel  TimeDomain=Discrete-time  UseExternalTs=off  SampleTime=0.005  IntegratorMethod=Backward Euler  FilterMethod=Forward Euler  ControllerParametersSource=external  P=1  I=1  UseKiTs=on  D=0  N=100  UseFilter=off  TunerSelectOption=Transfer Function Based (PID Tuner App)  InitialConditionSource=internal  InitialConditionForIntegrator=0  InitialConditionForFilter=0  DifferentiatorICPrevScaledInput=0  ExternalReset=rising  TrackingMode=off  Kt=1  LimitOutput=on  SatLimitsSource=internal  UpperSaturationLimit=80000  LowerSaturationLimit=0  LinearizeAsGain=on  AntiWindupMode=clamping  Kb=2  SaturateOnIntegerOverflow=on  POutMin=[]  POutMax=[]  IOutMin=[]  IOutMax=[]  DOutMin=[]  DOutMax=[]  NOutMin=[]  NOutMax=[]  SumOutMin=[]  SumOutMax=[]  SaturationOutMin=[]  SaturationOutMax=[]  PParamMin=[]  PParamMax=[]  IParamMin=[]  IParamMax=[]  DParamMin=[]  DParamMax=[]  NParamMin=[]  NParamMax=[]  KbParamMin=[]  KbParamMax=[]  KtParamMin=[]  KtParamMax=[]  KbOutMin=[]  KbOutMax=[]  KtOutMin=[]  KtOutMax=[]  IntegratorOutMin=[]  IntegratorOutMax=[]  FilterOutMin=[]  FilterOutMax=[]  SumI1OutMin=[]  SumI1OutMax=[]  SumI2OutMin=[]  SumI2OutMax=[]  SumI3OutMin=[]  SumI3OutMax=[]  SumI4OutMin=[]  SumI4OutMax=[]  SumDOutMin=[]  SumDOutMax=[]  DifferentiatorOutMin=[]  DifferentiatorOutMax=[]  FilterDiffOutCoefMin=[]  FilterDiffOutCoefMax=[]  ReciprocalOutMin=[]  ReciprocalOutMax=[]  SumDenOutMin=[]  SumDenOutMax=[]  SumNumOutMin=[]  SumNumOutMax=[]  DivideOutMin=[]  DivideOutMax=[]  UdiffTsProdOutMin=[]  UdiffTsProdOutMax=[]  NTsProdOutMin=[]  NTsProdOutMax=[]  UintegralTsProdOutMin=[]  UintegralTsProdOutMax=[]  UngainTsProdOutMin=[]  UngainTsProdOutMax=[]  ClampingZeroOutDataTypeStr=Inherit: Inherit via back propagation  ClampingZeroOutMin=[]  ClampingZeroOutMax=[]  FilterDenConstantOutDataTypeStr=Inherit: Inherit via back propagation  FilterDenConstantOutMin=[]  FilterDenConstantOutMax=[]  PCopyOutDataTypeStr=Inherit: Inherit via back propagation  PCopyOutMin=[]  PCopyOutMax=[]  NCopyOutDataTypeStr=Inherit: Inherit via back propagation  NCopyOutMin=[]  NCopyOutMax=[]  IntegratorContinuousStateAttributes=''  IntegratorStateMustResolveToSignalObject=off  IntegratorRTWStateStorageClass=Auto  FilterContinuousStateAttributes=''  FilterStateMustResolveToSignalObject=off  FilterRTWStateStorageClass=Auto  ParallelPVariant=ExternalParameters  IdealPVariant=Disabled  IVariant=ExternalParameters  DVariant=ExternalParameters  IntegratorVariant=Discrete  SatVariant=Enabled  AWVariant=DiscClampingParallel  PCopyVariant=Disabled  TRVariant=Disabled  FdbkBlocksVariant=Feedback  IdealPFdbkVariant=Passthrough  SatFdbkVariant=Passthrough  DerivativeFilterVariant=Differentiator  NVariant=Passthrough  NCopyVariant=Disabled_SignalSpec  FilterICVariant=InternalICsDifferentiator  IntegratorICVariant=InternalICs  ExternalResetVariant=ExternalReset  TRSumVariant=Passthrough  SumFdbkVariant=Enabled  SumVariant=Sum_PID  TsampFilterVariant=InternalTs  TsampNgainVariant=Passthrough  TsampIntegralVariant=Passthrough  ExternalSaturationOutDataTypeStr=Inherit: Same as second input  aMode=0
  PReductionTotal : Outport
  wires:
  PID Controller/1 -> PReductionTotal/1  "control input delta_P"
  D_PC/1 -> PID Controller/4
  P_PC/1 -> PID Controller/2
  PError/1 -> PID Controller/1
  I_PC/1 -> PID Controller/3
  ResetPID_PC/1 -> PID Controller/5
